simulink model "SoftStopper"  (R2016b)
settings: Solver=FixedStepDiscrete  StartTime=0.0  StopTime=inf  FixedStep=0.002  RelTol=1e-3  EnableMultiTasking=on
settings Model: xpc_rtwmakecfg_data=_xpcethercatlib_  Creator=march  LastModifiedBy=march
settings SolverCC: EnableConcurrentExecution=on  AutoInsertRateTranBlk=on
settings DataIOCC: SaveFormat=StructureWithTime  SaveOutput=off  SaveTime=off
settings OptimizationCC: BlockReduction=off  OptimizeBlockIOStorage=off  BufferReuse=off  GlobalBufferReuse=off  ExpressionFolding=off  LocalBlockOutputs=off
settings HardwareCC: ProdBitPerPointer=32  ProdBitPerSizeT=32  ProdBitPerPtrDiffT=32  ProdLargestAtomicFloat=None  ProdWordSize=32  ProdLongLongMode=on  ProdHWDeviceType=Generic->32-bit x86 compatible
settings RTWCC: SystemTargetFile=slrt.tlc  TemplateMakefile=slrt_default_tmf  PostCodeGenCommand=SomanetTuning_make_rtw_hook  Description=Simulink Real-Time  RTWVerbose=off  CodeExecutionProfiling=on  RTWCompilerOptimization=on
settings SimulinkRealTimeCC: xPCModelTimeoutSecs=20

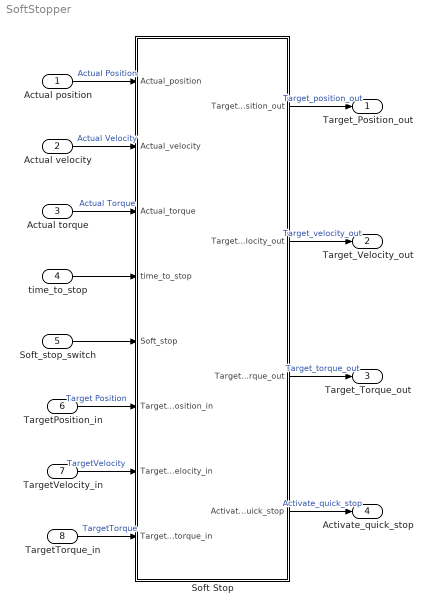
== system SoftStopper ==
  Actual position : Inport  OutDataTypeStr=int32  PortDimensions=1  SampleTime=[0.002,0]
  Actual velocity : Inport  Port=2  OutDataTypeStr=int32  PortDimensions=1  SampleTime=[0.002,0]
  Actual torque : Inport  Port=3  OutDataTypeStr=int16  PortDimensions=1  SampleTime=[0.002,0]
  time_to_stop : Inport  Port=4  OutDataTypeStr=double  PortDimensions=1  SampleTime=0.002
  Soft_stop_switch : Inport  Port=5  OutDataTypeStr=double  PortDimensions=1  SampleTime=0.002
  TargetPosition_in : Inport  Port=6  OutDataTypeStr=int32  PortDimensions=1  SampleTime=[0.002,0]
  TargetVelocity_in : Inport  Port=7  OutDataTypeStr=int32  PortDimensions=1  SampleTime=[0.002,0]
  TargetTorque_in : Inport  Port=8  OutDataTypeStr=int16  PortDimensions=1  SampleTime=[0.002,0]
  Soft Stop : MATLAB Function  TreatAsAtomicUnit=on
  Target_Position_out : Outport  OutDataTypeStr=int32  PortDimensions=1  SampleTime=[0.002,0]
  Target_Velocity_out : Outport  Port=2  OutDataTypeStr=int32  PortDimensions=1  SampleTime=[0.002,0]
  Target_Torque_out : Outport  Port=3  OutDataTypeStr=int16  PortDimensions=1  SampleTime=[0.002,0]
  Activate_quick_stop : Outport  Port=4  OutDataTypeStr=boolean  PortDimensions=1  SampleTime=[0.002,0]
  wires:
  Actual velocity/1 -> Soft Stop/2(Actual_velocity)  "Actual Velocity"
  Soft_stop_switch/1 -> Soft Stop/5(Soft_stop)
  Actual position/1 -> Soft Stop/1(Actual_position)  "Actual Position"
  Actual torque/1 -> Soft Stop/3(Actual_torque)  "Actual Torque"
  time_to_stop/1 -> Soft Stop/4(time_to_stop)
  Soft Stop/1(Target_position_out) -> Target_Position_out/1  "Target_position_out"
  Soft Stop/2(Target_velocity_out) -> Target_Velocity_out/1  "Target_velocity_out"
  Soft Stop/3(Target_torque_out) -> Target_Torque_out/1  "Target_torque_out"
  Soft Stop/4(Activate_quick_stop) -> Activate_quick_stop/1  "Activate_quick_stop"
  TargetVelocity_in/1 -> Soft Stop/7(Target_velocity_in)  "TargetVelocity"
  TargetPosition_in/1 -> Soft Stop/6(Target_position_in)  "Target Position"
  TargetTorque_in/1 -> Soft Stop/8(Target_torque_in)  "TargetTorque"

== matlab function SoftStopper/Soft Stop ==
  data: Actual_position input; Actual_velocity input; Actual_torque input; time_to_stop input; Soft_stop input; Target_position_in input; Target_velocity_in input; Target_position_out output; Target_velocity_out output; Target_torque_out output; Target_torque_in input; Activate_quick_stop output
% "Soft" Stop

%Should stop the motor smoothly within whilst not moving further then a
%certain max angle.

function [Target_position_out, Target_velocity_out, Target_torque_out, Activate_quick_stop] = ... 
    Soft_stop( Actual_position, Actual_velocity, Actual_torque, time_to_stop, Soft_stop, Target_position_in, Target_velocity_in, Target_torque_in)

persistent original_velocity
persistent original_torque
persistent count



if isempty(original_velocity)
    original_velocity   = int32(0);
    original_torque     = int16(0);
    count               = 0;
    
end


    
if Soft_stop ~= 0 || count ~= 0
    
    if count == 0
            %first time soft stop is activated it remembers the velocity
            %and torque it was on
            
            original_velocity = Actual_velocity;
            original_torque   = Actual_torque;
    end
    
    %Reduces the target setpoint to zero pos/vel/tor within time_to_stop
    Target_torque_out = int16(original_torque) - int16(original_torque /1.5);
    Target_velocity_out = int32(original_velocity) - int32(original_velocity /(time_to_stop / 0.002)) ;
    Target_position_out = int32(Actual_position);
    
    count = count +1;
    Activate_quick_stop = true;
else
    
    
    %does not affect target points when soft stop is not activated
     Target_velocity_out = Target_velocity_in;
     Target_position_out = Target_position_in;
     Target_torque_out   = Target_torque_in;
     Activate_quick_stop = false;
    
end

%puts on quick-stop when soft_stop is completed and reset the soft_stop
%switch

if count == time_to_stop/0.002
    
    %makes sure setpoints actually are zero at end of the soft_stop
    Target_torque_out =int16(0);
    Target_velocity_out = int32(0);
   
    count = 0;
    
end

    
end
